simulink model "Discrete_EKF_2FMU"  (R2022a)
settings: Solver=ode23s  StartTime=0.0  StopTime=10  RelTol=1e-3
settings Model: Creator=au707539  LastModifiedBy=au707539
settings SolverCC: MaxZcPerStep=1
settings DebuggingCC: UnderSpecifiedDimensionMsg=warning

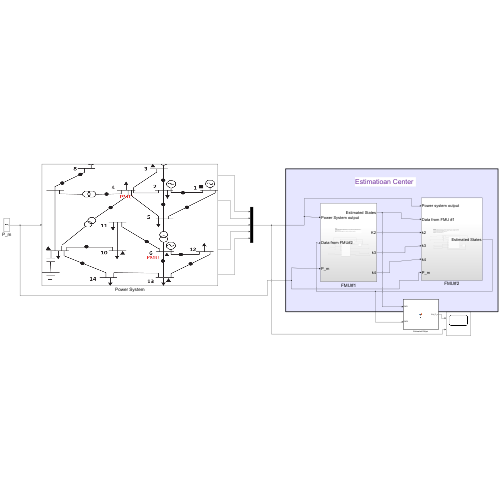
[thumbnail: Simulink's stored preview of the top-level diagram]
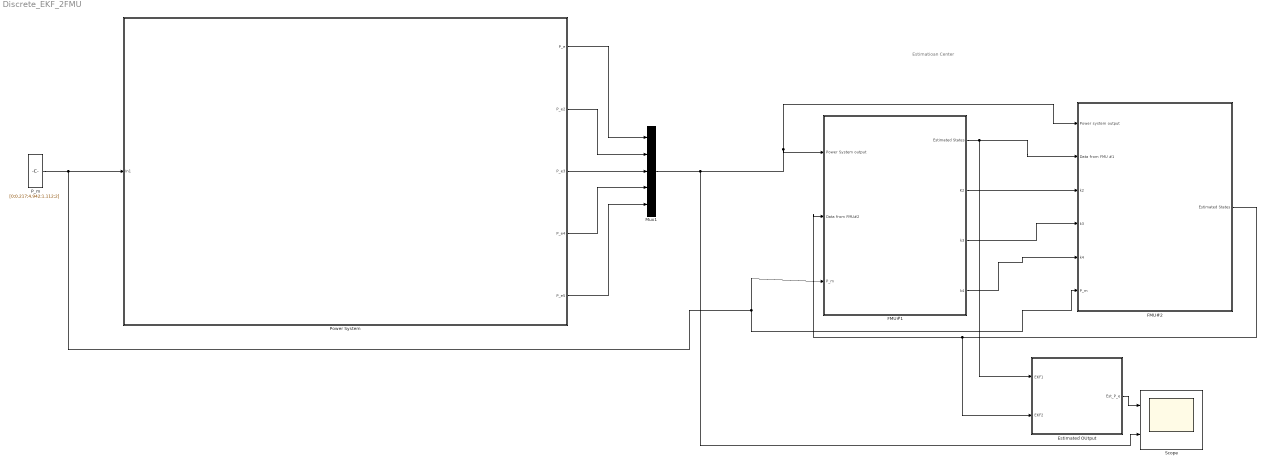
== system Discrete_EKF_2FMU ==
  note: Estimatioan Center
  Estimated OUtput : MATLAB Function  TreatAsAtomicUnit=on
  FMU#1 : Subsystem
  FMU#2 : Subsystem
  Mux1 : Mux  Inputs=5
  P_m : Constant  Value=[0;0.217;4.942;1.112;2]
  Power System : Subsystem
      mask Display: image('IEEE.png'); % Use "Edit Image" on toolstrip to change.
  Scope : Scope  NumInputPorts=2
  wires:
  P_m/1 -> FMU#1/3(P_m), FMU#2/6(P_m), Power System/1(In1)
  Mux1/1 -> Scope/2, FMU#2/1(Power system output), FMU#1/1(Power System output)
  Power System/1(P_e) -> Mux1/1
  Power System/2(P_e2) -> Mux1/2
  Power System/3(P_e3) -> Mux1/3
  Power System/4(P_e4) -> Mux1/4
  Power System/5(P_e5) -> Mux1/5
  FMU#1/1(Estimated States) -> Estimated OUtput/1(EKF1), FMU#2/2(Data from FMU #1)
  FMU#1/2(K2) -> FMU#2/3(k2)
  FMU#1/3(k3) -> FMU#2/4(k3)
  FMU#1/4(k4) -> FMU#2/5(k4)
  FMU#2/1(Estimated States) -> Estimated OUtput/2(EKF2), FMU#1/2(Data from FMU#2)
  Estimated OUtput/1(Est_P_e) -> Scope/1

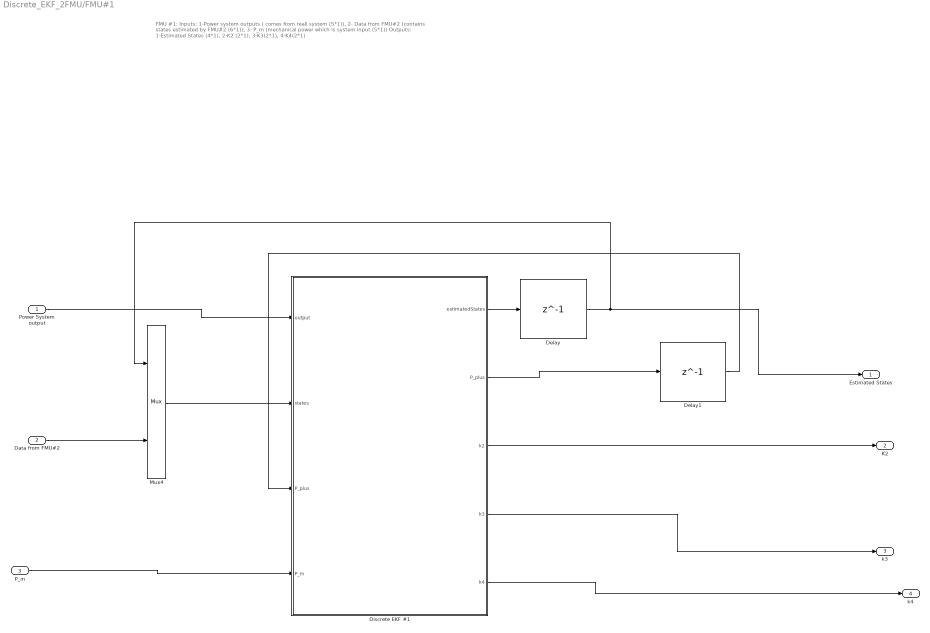
== system Discrete_EKF_2FMU/FMU#1 ==
  note: FMU #1:
      | Inputs: 1-Power system outputs ( comes from reall system (5*1)), 2- Data from FMU#2 (contains states estimated by FMU#2 (6*1)), 3- P_m (mechanical power which is system input (5*1))
      | Outputs: 1-Estimated States (4*1), 2-K2 (2*1), 3-K3(2*1), 4-K4(2*1)
  Power System output : Inport
  Data from FMU#2 : Inport  Port=2
  P_m : Inport  Port=3
  Delay : Delay  DelayLength=1  InitialCondition=[-0.152730000000000,-0.230910000000000,1,1]'  SampleTime=1e-4
  Delay1 : Delay  DelayLength=1  InitialCondition=0.01*eye(4)  SampleTime=1e-4
  Discrete EKF #1 : MATLAB Function  TreatAsAtomicUnit=on
  Mux4 : Mux  Inputs=2
  Estimated States : Outport
  K2 : Outport  Port=2
  k3 : Outport  Port=3
  k4 : Outport  Port=4
  wires:
  Discrete EKF #1/2(P_plus) -> Delay1/1
  Discrete EKF #1/1(estimatedStates) -> Delay/1
  Discrete EKF #1/3(k2) -> K2/1
  Power System output/1 -> Discrete EKF #1/1(output)
  Delay/1 -> Mux4/1, Estimated States/1
  Discrete EKF #1/4(k3) -> k3/1
  Mux4/1 -> Discrete EKF #1/2(states)
  Delay1/1 -> Discrete EKF #1/3("P_plus ")
  Discrete EKF #1/5(k4) -> k4/1
  P_m/1 -> Discrete EKF #1/4(P_m)
  Data from FMU#2/1 -> Mux4/2

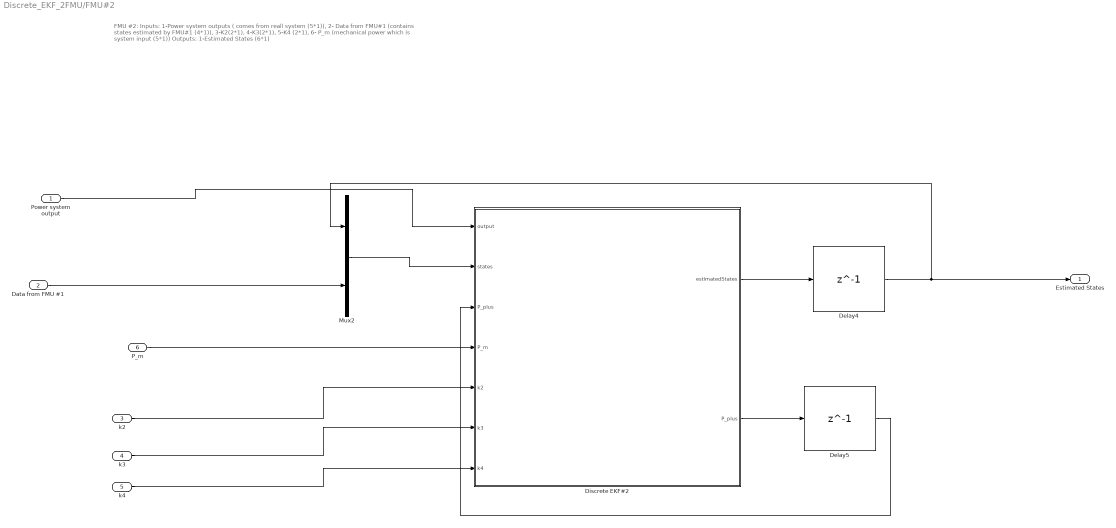
== system Discrete_EKF_2FMU/FMU#2 ==
  note: FMU #2:
      | Inputs: 1-Power system outputs ( comes from reall system (5*1)), 2- Data from FMU#1 (contains states estimated by FMU#1 (4*1)), 3-K2(2*1), 4-K3(2*1), 5-K4 (2*1), 6- P_m (mechanical power which is system input (5*1))
      | Outputs: 1-Estimated States (6*1)
  Power system output : Inport
  Data from FMU #1 : Inport  Port=2
  k2 : Inport  Port=3
  k3 : Inport  Port=4
  k4 : Inport  Port=5
  P_m : Inport  Port=6
  Delay4 : Delay  DelayLength=1  InitialCondition=[1.07618884220704,0.179610235169918,-0.222670000000000,1,1,1]'  SampleTime=1e-4
  Delay5 : Delay  DelayLength=1  InitialCondition=0.01*eye(6)  SampleTime=1e-4
  Discrete EKF#2 : MATLAB Function  TreatAsAtomicUnit=on
  Mux2 : Mux  Inputs=2
  Estimated States : Outport
  wires:
  Delay4/1 -> Mux2/1, Estimated States/1
  Data from FMU #1/1 -> Mux2/2
  Discrete EKF#2/1(estimatedStates) -> Delay4/1
  Delay5/1 -> Discrete EKF#2/3("P_plus ")
  Discrete EKF#2/2(P_plus) -> Delay5/1
  Mux2/1 -> Discrete EKF#2/2(states)
  P_m/1 -> Discrete EKF#2/4(P_m)
  Power system output/1 -> Discrete EKF#2/1(output)
  k4/1 -> Discrete EKF#2/7(k4)
  k2/1 -> Discrete EKF#2/5(k2)
  k3/1 -> Discrete EKF#2/6(k3)

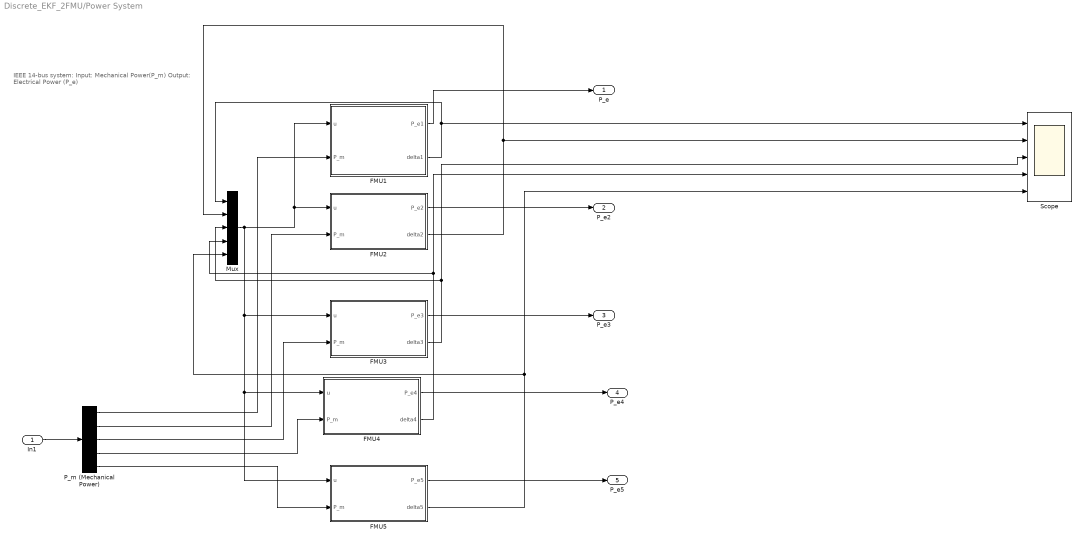
== system Discrete_EKF_2FMU/Power System ==
  note: IEEE 14-bus system:
      | Input: Mechanical Power(P_m)
      | Output: Electrical Power (P_e)
  In1 : Inport
  FMU1 : Subsystem
  FMU2 : Subsystem
  FMU3 : Subsystem
  FMU4 : Subsystem
  FMU5 : Subsystem
  Mux : Mux  Inputs=5
  P_m (Mechanical Power) : Demux  Outputs=5
  Scope : Scope  NumInputPorts=5
  P_e : Outport
  P_e2 : Outport  Port=2
  P_e3 : Outport  Port=3
  P_e4 : Outport  Port=4
  P_e5 : Outport  Port=5
  wires:
  FMU1/2(delta1) -> Scope/1, Mux/1
  FMU2/2(delta2) -> Scope/2, Mux/2
  In1/1 -> P_m (Mechanical Power)/1
  P_m (Mechanical Power)/1 -> FMU1/2(P_m)
  FMU1/1(P_e1) -> P_e/1
  P_m (Mechanical Power)/2 -> FMU2/2(P_m)
  FMU2/1(P_e2) -> P_e2/1
  P_m (Mechanical Power)/3 -> FMU3/2(P_m)
  FMU3/2(delta3) -> Scope/3, Mux/3
  FMU3/1(P_e3) -> P_e3/1
  P_m (Mechanical Power)/4 -> FMU4/2(P_m)
  FMU4/2(delta4) -> Scope/4, Mux/4
  FMU4/1(P_e4) -> P_e4/1
  P_m (Mechanical Power)/5 -> FMU5/2(P_m)
  FMU5/1(P_e5) -> P_e5/1
  FMU5/2(delta5) -> Mux/5, Scope/5
  Mux/1 -> FMU5/1(u), FMU4/1(u), FMU3/1(u), FMU2/1(u), FMU1/1(u)

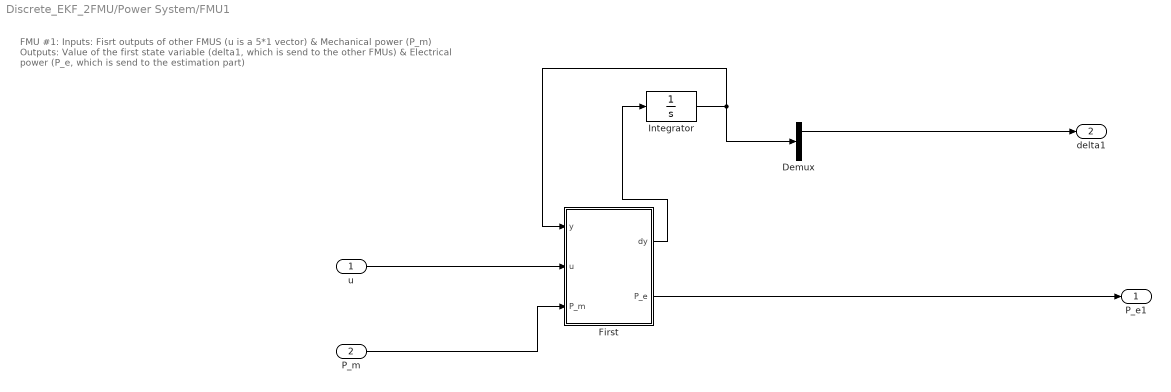
== system Discrete_EKF_2FMU/Power System/FMU1 ==
  note: FMU #1:
      | Inputs: Fisrt outputs of other FMUS (u is a 5*1 vector) & Mechanical power (P_m)
      | Outputs: Value of the first state variable (delta1, which is send to the other FMUs) & Electrical power (P_e, which is send to the estimation part)
  u : Inport
  P_m : Inport  Port=2
  Demux : Demux  Outputs=2
  First : MATLAB Function  TreatAsAtomicUnit=on
  Integrator : Integrator  InitialCondition=[1.0762;1]
  P_e1 : Outport
  delta1 : Outport  Port=2
  wires:
  u/1 -> First/2(u)
  Integrator/1 -> First/1(y), Demux/1
  First/1(dy) -> Integrator/1
  P_m/1 -> First/3(P_m)
  First/2(P_e) -> P_e1/1
  Demux/1 -> delta1/1

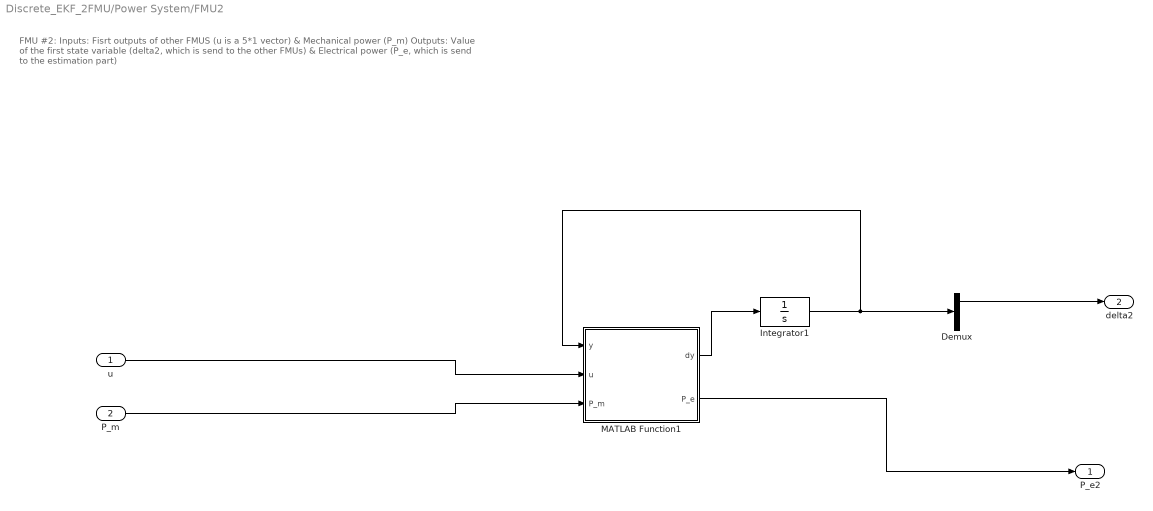
== system Discrete_EKF_2FMU/Power System/FMU2 ==
  note: FMU #2:
      | Inputs: Fisrt outputs of other FMUS (u is a 5*1 vector) & Mechanical power (P_m)
      | Outputs: Value of the first state variable (delta2, which is send to the other FMUs) & Electrical power (P_e, which is send to the estimation part)
  u : Inport
  P_m : Inport  Port=2
  Demux : Demux  Outputs=2
  Integrator1 : Integrator  InitialCondition=[0.1796;1]
  MATLAB Function1 : MATLAB Function  TreatAsAtomicUnit=on
  P_e2 : Outport
  delta2 : Outport  Port=2
  wires:
  P_m/1 -> MATLAB Function1/3(P_m)
  MATLAB Function1/1(dy) -> Integrator1/1
  u/1 -> MATLAB Function1/2(u)
  Integrator1/1 -> Demux/1, MATLAB Function1/1(y)
  Demux/1 -> delta2/1
  MATLAB Function1/2(P_e) -> P_e2/1

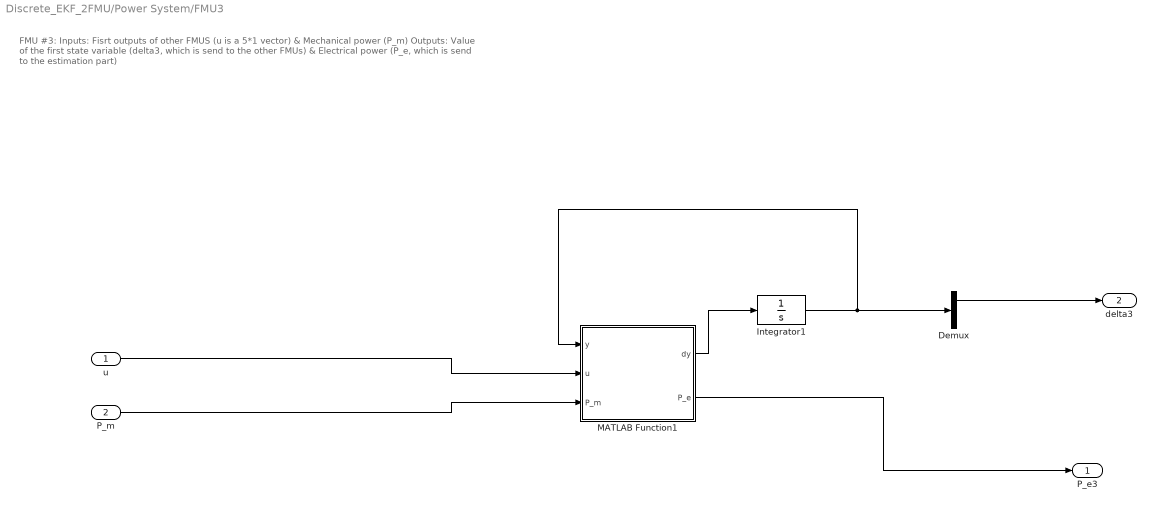
== system Discrete_EKF_2FMU/Power System/FMU3 ==
  note: FMU #3:
      | Inputs: Fisrt outputs of other FMUS (u is a 5*1 vector) & Mechanical power (P_m)
      | Outputs: Value of the first state variable (delta3, which is send to the other FMUs) & Electrical power (P_e, which is send to the estimation part)
  u : Inport
  P_m : Inport  Port=2
  Demux : Demux  Outputs=2
  Integrator1 : Integrator  InitialCondition=[-0.22267;1]
  MATLAB Function1 : MATLAB Function  TreatAsAtomicUnit=on
  P_e3 : Outport
  delta3 : Outport  Port=2
  wires:
  P_m/1 -> MATLAB Function1/3(P_m)
  MATLAB Function1/1(dy) -> Integrator1/1
  u/1 -> MATLAB Function1/2(u)
  Integrator1/1 -> Demux/1, MATLAB Function1/1(y)
  Demux/1 -> delta3/1
  MATLAB Function1/2(P_e) -> P_e3/1

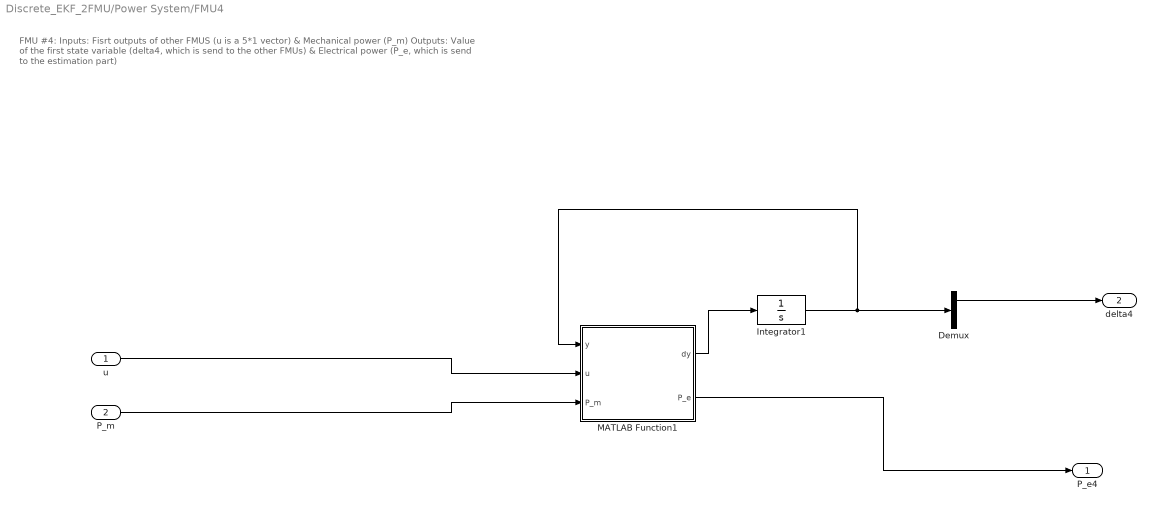
== system Discrete_EKF_2FMU/Power System/FMU4 ==
  note: FMU #4:
      | Inputs: Fisrt outputs of other FMUS (u is a 5*1 vector) & Mechanical power (P_m)
      | Outputs: Value of the first state variable (delta4, which is send to the other FMUs) & Electrical power (P_e, which is send to the estimation part)
  u : Inport
  P_m : Inport  Port=2
  Demux : Demux  Outputs=2
  Integrator1 : Integrator  InitialCondition=[-0.15273;1]
  MATLAB Function1 : MATLAB Function  TreatAsAtomicUnit=on
  P_e4 : Outport
  delta4 : Outport  Port=2
  wires:
  P_m/1 -> MATLAB Function1/3(P_m)
  MATLAB Function1/1(dy) -> Integrator1/1
  u/1 -> MATLAB Function1/2(u)
  Integrator1/1 -> Demux/1, MATLAB Function1/1(y)
  Demux/1 -> delta4/1
  MATLAB Function1/2(P_e) -> P_e4/1

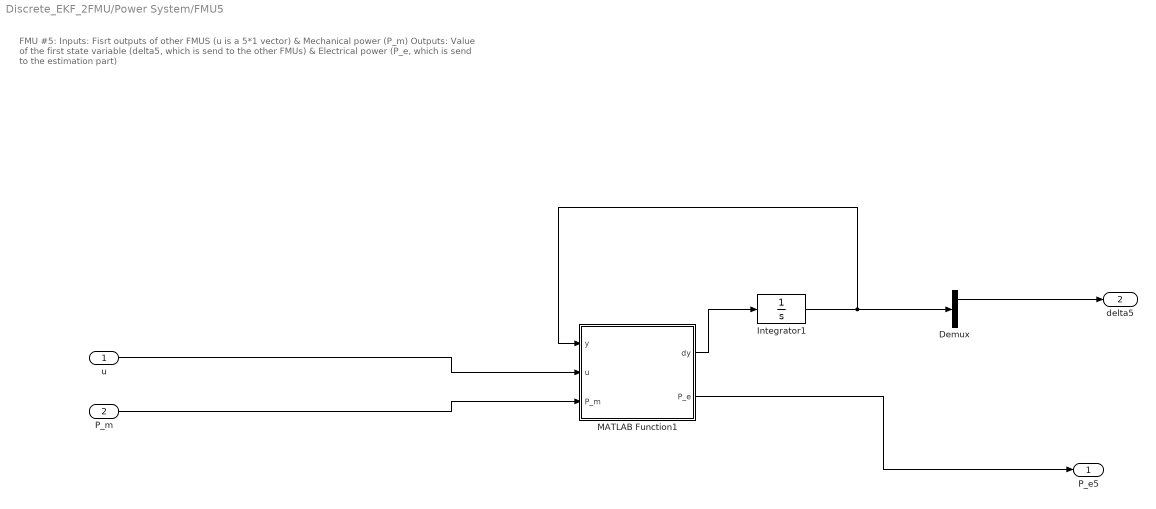
== system Discrete_EKF_2FMU/Power System/FMU5 ==
  note: FMU #5:
      | Inputs: Fisrt outputs of other FMUS (u is a 5*1 vector) & Mechanical power (P_m)
      | Outputs: Value of the first state variable (delta5, which is send to the other FMUs) & Electrical power (P_e, which is send to the estimation part)
  u : Inport
  P_m : Inport  Port=2
  Demux : Demux  Outputs=2
  Integrator1 : Integrator  InitialCondition=[-0.23091;1]
  MATLAB Function1 : MATLAB Function  TreatAsAtomicUnit=on
  P_e5 : Outport
  delta5 : Outport  Port=2
  wires:
  P_m/1 -> MATLAB Function1/3(P_m)
  MATLAB Function1/1(dy) -> Integrator1/1
  u/1 -> MATLAB Function1/2(u)
  Integrator1/1 -> Demux/1, MATLAB Function1/1(y)
  Demux/1 -> delta5/1
  MATLAB Function1/2(P_e) -> P_e5/1

== matlab function Discrete_EKF_2FMU/Power System/FMU2/MATLAB Function1 ==
  data: y input; u input; dy output; P_m input; P_e output
%% This function formulates the dynamic model of the second synchronous machine in IEEE-14 bus test system
%% y is the state vector related to this Genrator, u is vector of all generators angles (delta), and P-m is Mechanical power injected to this machine
%% dy is the derivative of y which is calculated in this function and P-e is the electrical power which is calculated in this function
function [dy,P_e] = fcn(y,u,P_m)
dy=zeros(2,1);
P_e=0;
%%%%%%%Generators and network parameters (they can be defined as global
%%%%%%%parameters because they are fixed for all generators)%%%%%%%%%%%
N_SG=5;
X_d=[0.898 1.05 1.05 1.25 1.25];
Vol_mag=[1.06 1.045 1.01 1.011981 1.049336 1.016012 1.07 1.09 1.032756 1.03177 1.04708 1.053428 1.046967 1.020701];
P_Gen=[2.32 0.4 0 0 0];
Q_Gen=[0 0.424 0 0 0];
VOl_mag_Gen=[Vol_mag(1) Vol_mag(2) Vol_mag(3) Vol_mag(6) Vol_mag(8)];
M=[3.52e-3 0.436e-3 0.436e-3 1.406e-4 1.406e-4];
D=[2 2 2 2 2];
Y=[0.1017-2.4199i, 0.0096+0.9097i, -0.0567+0.5006i, -0.0322+0.4973i, -0.0186+0.5531i; 0.0096+0.9097i, 0.1375-3.5521i, -0.0574+0.9568i, -0.0437+0.8608i, ...
    -0.0395+0.8903i; -0.0567+0.5006i, -0.0574+0.9568i, 0.2630-2.9134i, -0.0640+0.8148i, -0.0791+0.6968i; -0.0322+0.4973i, -0.0437+0.8608i, -0.0640+0.8148i,...
    0.1156-3.0762i, 0.0303+0.9547i; -0.0186+0.5531i, -0.0395+0.8903i, -0.0791+0.6968i, 0.0303+0.9547i, 0.1117-3.0513i];
% [v_r, v_i]=pol2cart(Degrre_Gen,Vol_mag_Gen);

E_abs=zeros(5,1);
for i=1:5
    %     delta0(i)=angle(VOl_mag_Gen(i)+Q_Gen(i).*X_d(i)./VOl_mag_Gen(i) + 1i*P_Gen(i).*X_d(i)./VOl_mag_Gen(i))+Degrre_Gen(i);
    E_abs(i)=abs(VOl_mag_Gen(i)+Q_Gen(i).*X_d(i)./VOl_mag_Gen(i) + 1i*P_Gen(i).*X_d(i)./VOl_mag_Gen(i));
end
%%%%%%%%%%%%%%%%%%%%%%%%%%
delta=u(1:5);
sum1=0; %% local parameter
for j=1:N_SG

    sum1=sum1+E_abs(2)*E_abs(j)*abs(Y(2,j))*cos(delta(2)-delta(j)-angle(Y(2,j))); % All angles in Radian
end
P_e=sum1;

P_e=sum1;  % Second output (which is send to the estimation part)

dy(1)=y(2); %first entry of the function output

dy(2) =(1/M(2))*(P_m-P_e-D(2)*y(2));  %Second entry of the function output

== matlab function Discrete_EKF_2FMU/Power System/FMU1/First ==
  data: y input; u input; dy output; P_m input; P_e output
%% This function formulates the dynamic model of the first synchronous machine in IEEE-14 bus test system
%% y is the state vector related to this Genrator, u is vector of all generators angles (delta), and P-m is Mechanical power injected to this machine
%% dy is the derivative of y which is calculated in this function and P-e is the electrical power which is calculated in this function
function [dy,P_e] = fcn(y,u,P_m) 
dy=zeros(2,1);

%%%%%%%Generators and network parameters (they can be defined as global
%%%%%%%parameters because they are fixed for all generators)%%%%%%%%%%%%%
N_SG=5;
X_d=[0.898 1.05 1.05 1.25 1.25];
Vol_mag=[1.06 1.045 1.01 1.011981 1.049336 1.016012 1.07 1.09 1.032756 1.03177 1.04708 1.053428 1.046967 1.020701];
P_Gen=[2.32 0.4 0 0 0];
Q_Gen=[0 0.424 0 0 0];
VOl_mag_Gen=[Vol_mag(1) Vol_mag(2) Vol_mag(3) Vol_mag(6) Vol_mag(8)];
M=[3.52e-3 0.436e-3 0.436e-3 1.406e-4 1.406e-4];
D=[2 2 2 2 2];
Y=[0.1017-2.4199i, 0.0096+0.9097i, -0.0567+0.5006i, -0.0322+0.4973i, -0.0186+0.5531i; 0.0096+0.9097i, 0.1375-3.5521i, -0.0574+0.9568i, -0.0437+0.8608i, ...
    -0.0395+0.8903i; -0.0567+0.5006i, -0.0574+0.9568i, 0.2630-2.9134i, -0.0640+0.8148i, -0.0791+0.6968i; -0.0322+0.4973i, -0.0437+0.8608i, -0.0640+0.8148i,...
    0.1156-3.0762i, 0.0303+0.9547i; -0.0186+0.5531i, -0.0395+0.8903i, -0.0791+0.6968i, 0.0303+0.9547i, 0.1117-3.0513i];
% [v_r, v_i]=pol2cart(Degrre_Gen,Vol_mag_Gen);

E_abs=zeros(5,1); %local parameter
for i=1:5
    %     delta0(i)=angle(VOl_mag_Gen(i)+Q_Gen(i).*X_d(i)./VOl_mag_Gen(i) + 1i*P_Gen(i).*X_d(i)./VOl_mag_Gen(i))+Degrre_Gen(i);
    E_abs(i)=abs(VOl_mag_Gen(i)+Q_Gen(i).*X_d(i)./VOl_mag_Gen(i) + 1i*P_Gen(i).*X_d(i)./VOl_mag_Gen(i));
end
%%%%%%%%%%%%%%%%%%%%%%%%%%
delta=u(1:5);
sum1=0; %% local parameter
for j=1:N_SG

    sum1=sum1+E_abs(1)*E_abs(j)*abs(Y(1,j))*cos(delta(1)-delta(j)-angle(Y(1,j))); % All angles in Radian
end

P_e=sum1;  % Second output (which is send to the estimation part)

dy(1)=y(2); %first entry of the function output

dy(2) =(1/M(1))*(P_m-P_e-D(1)*y(2)); %Second entry of the function output

== matlab function Discrete_EKF_2FMU/Power System/FMU4/MATLAB Function1 ==
  data: y input; u input; dy output; P_m input; P_e output
%% This function formulates the dynamic model of the fourth synchronous machine in IEEE-14 bus test system
%% y is the state vector related to this Genrator, u is vector of all generators angles (delta), and P-m is Mechanical power injected to this machine
%% dy is the derivative of y which is calculated in this function and P-e is the electrical power which is calculated in this function
function [dy,P_e] = fcn(y,u,P_m)
dy=zeros(2,1);
P_e=0;
%%%%%%%Generators and network parameters (they can be defined as global
%%%%%%%parameters because they are fixed for all generators)%%%%%%%%%%%
N_SG=5;
X_d=[0.898 1.05 1.05 1.25 1.25];
Vol_mag=[1.06 1.045 1.01 1.011981 1.049336 1.016012 1.07 1.09 1.032756 1.03177 1.04708 1.053428 1.046967 1.020701];
P_Gen=[2.32 0.4 0 0 0];
Q_Gen=[0 0.424 0 0 0];
VOl_mag_Gen=[Vol_mag(1) Vol_mag(2) Vol_mag(3) Vol_mag(6) Vol_mag(8)];
M=[3.52e-3 0.436e-3 0.436e-3 1.406e-4 1.406e-4];
D=[2 2 2 2 2];
Y=[0.1017-2.4199i, 0.0096+0.9097i, -0.0567+0.5006i, -0.0322+0.4973i, -0.0186+0.5531i; 0.0096+0.9097i, 0.1375-3.5521i, -0.0574+0.9568i, -0.0437+0.8608i, ...
    -0.0395+0.8903i; -0.0567+0.5006i, -0.0574+0.9568i, 0.2630-2.9134i, -0.0640+0.8148i, -0.0791+0.6968i; -0.0322+0.4973i, -0.0437+0.8608i, -0.0640+0.8148i,...
    0.1156-3.0762i, 0.0303+0.9547i; -0.0186+0.5531i, -0.0395+0.8903i, -0.0791+0.6968i, 0.0303+0.9547i, 0.1117-3.0513i];
% [v_r, v_i]=pol2cart(Degrre_Gen,Vol_mag_Gen);

E_abs=zeros(5,1);
for i=1:5
    %     delta0(i)=angle(VOl_mag_Gen(i)+Q_Gen(i).*X_d(i)./VOl_mag_Gen(i) + 1i*P_Gen(i).*X_d(i)./VOl_mag_Gen(i))+Degrre_Gen(i);
    E_abs(i)=abs(VOl_mag_Gen(i)+Q_Gen(i).*X_d(i)./VOl_mag_Gen(i) + 1i*P_Gen(i).*X_d(i)./VOl_mag_Gen(i));
end
%%%%%%%%%%%%%%%%%%%%%%%%%%
delta=u(1:5);
sum1=0; %% local parameter
for j=1:N_SG

    sum1=sum1+E_abs(4)*E_abs(j)*abs(Y(4,j))*cos(delta(4)-delta(j)-angle(Y(4,j))); % All angles in Radian
end

P_e=sum1;

P_e=sum1;  % Second output (which is send to the estimation part)

dy(1)=y(2); %first entry of the function output

dy(2) =(1/M(4))*(P_m-P_e-D(4)*y(2));  %Second entry of the function output

== matlab function Discrete_EKF_2FMU/Power System/FMU5/MATLAB Function1 ==
  data: y input; u input; dy output; P_m input; P_e output
%% This function formulates the dynamic model of the fifth synchronous machine in IEEE-14 bus test system
%% y is the state vector related to this Genrator, u is vector of all generators angles (delta), and P-m is Mechanical power injected to this machine
%% dy is the derivative of y which is calculated in this function and P-e is the electrical power which is calculated in this function
function [dy,P_e] = fcn(y,u,P_m)
dy=zeros(2,1);
P_e=0;
%%%%%%%Generators and network parameters (they can be defined as global
%%%%%%%parameters because they are fixed for all generators)%%%%%%%%%%%
N_SG=5;
X_d=[0.898 1.05 1.05 1.25 1.25];
Vol_mag=[1.06 1.045 1.01 1.011981 1.049336 1.016012 1.07 1.09 1.032756 1.03177 1.04708 1.053428 1.046967 1.020701];
P_Gen=[2.32 0.4 0 0 0];
Q_Gen=[0 0.424 0 0 0];
VOl_mag_Gen=[Vol_mag(1) Vol_mag(2) Vol_mag(3) Vol_mag(6) Vol_mag(8)];
M=[3.52e-3 0.436e-3 0.436e-3 1.406e-4 1.406e-4];
D=[2 2 2 2 2];
Y=[0.1017-2.4199i, 0.0096+0.9097i, -0.0567+0.5006i, -0.0322+0.4973i, -0.0186+0.5531i; 0.0096+0.9097i, 0.1375-3.5521i, -0.0574+0.9568i, -0.0437+0.8608i, ...
    -0.0395+0.8903i; -0.0567+0.5006i, -0.0574+0.9568i, 0.2630-2.9134i, -0.0640+0.8148i, -0.0791+0.6968i; -0.0322+0.4973i, -0.0437+0.8608i, -0.0640+0.8148i,...
    0.1156-3.0762i, 0.0303+0.9547i; -0.0186+0.5531i, -0.0395+0.8903i, -0.0791+0.6968i, 0.0303+0.9547i, 0.1117-3.0513i];
% [v_r, v_i]=pol2cart(Degrre_Gen,Vol_mag_Gen);

E_abs=zeros(5,1);
for i=1:5
    %     delta0(i)=angle(VOl_mag_Gen(i)+Q_Gen(i).*X_d(i)./VOl_mag_Gen(i) + 1i*P_Gen(i).*X_d(i)./VOl_mag_Gen(i))+Degrre_Gen(i);
    E_abs(i)=abs(VOl_mag_Gen(i)+Q_Gen(i).*X_d(i)./VOl_mag_Gen(i) + 1i*P_Gen(i).*X_d(i)./VOl_mag_Gen(i));
end
%%%%%%%%%%%%%%%%%%%%%%%%%%
delta=u(1:5);
sum1=0; %% local parameter
for j=1:N_SG

    sum1=sum1+E_abs(5)*E_abs(j)*abs(Y(5,j))*cos(delta(5)-delta(j)-angle(Y(5,j))); % All angles in Radian
end

P_e=sum1;

P_e=sum1;  % Second output (which is send to the estimation part)

dy(1)=y(2); %first entry of the function output

dy(2) =(1/M(5))*(P_m-P_e-D(5)*y(2));  %Second entry of the function output

== matlab function Discrete_EKF_2FMU/FMU#1/Discrete EKF #1 ==
  data: output input; estimatedStates output; P_plus output; states input; P_plus input; P_m input; k2 output; k3 output; k4 output
%% This function calculates the estimated states of the synchronous machines #4 and #5
%% Outputs are: estimatedStates (4*1), P_plus (updated covariance matix 4*4), k2 (second parameters of RungeKutta for 4th and 5th angles 2*1), k3 (third parameters of RungeKutta for 4th and 5th angles 2*1),
%% k4 (fourth parameters of RungeKutta for 4th and 5th angles 2*1). Inputs are: output (comes from power system 5*1), states(includes states of previous sample of this function + FMU#2 10*1),P_plus (updated covariance matrix of previous sample 4*4),
%% and P_m (Mechanical power which is input of power system 5*1)
function [estimatedStates,P_plus,k2,k3,k4] = fcn(output,states,P_plus,P_m)

%%% Initialization
delta_plus=zeros(5,1);
delta_plus(4:5,1)=states(1:2,:);
delta_plus(1:3,1)=states(5:7,1);
omega_plus=zeros(5,1);
omega_plus(1:3,1)=states(8:10,1);
omega_plus(4:5,1)=states(3:4,:);

sigma=1e-2; % variance
Q=sigma^2*eye(4); %Covariance matrix of process noise
R=sigma^2*eye(2); % Covariance matrix of measurement noise
Dt=1e-4; % DelatT, sample time for discretization

%%% Power system parameters %%%%%%%%%%%%
n=5; %Number of synchronous machines
X_d=[0.898 1.05 1.05 1.25 1.25];
Angle_rad=[0 -0.0871 -0.22267 -0.1785 -0.23091 -0.15273 -0.25161 -0.23091 -0.25853 -0.26223 -0.25897 -0.26645 -0.2671 -0.28018];%% Bus voltage phases (all are in rad)
Vol_mag=[1.06 1.045 1.01 1.011981 1.049336 1.016012 1.07 1.09 1.032756 1.03177 1.04708 1.053428 1.046967 1.020701];%% Bus voltage magnitudes
P_Gen=[2.32 0.4 0 0 0]; % Active power
Q_Gen=[0 0.424 0 0 0]; % Reactive Power
M=[3.52e-3 0.436e-3 0.436e-3 1.406e-4 1.406e-4];
D=[2 2 2 2 2];
VOl_mag_Gen=[Vol_mag(1) Vol_mag(2) Vol_mag(3) Vol_mag(6) Vol_mag(8)];

%%Calculating the phases and magnitudes of the generator voltages
E_abs=zeros(5,1);
for i=1:5
    E_abs(i)=abs(VOl_mag_Gen(i)+Q_Gen(i).*X_d(i)./VOl_mag_Gen(i) + 1i*P_Gen(i).*X_d(i)./VOl_mag_Gen(i));
end

% Reduced admittance matrix (all in p.u.)
Y=[0.1017-2.4199i, 0.0096+0.9097i, -0.0567+0.5006i, -0.0322+0.4973i, -0.0186+0.5531i; 0.0096+0.9097i, 0.1375-3.5521i, -0.0574+0.9568i, -0.0437+0.8608i, ...
    -0.0395+0.8903i; -0.0567+0.5006i, -0.0574+0.9568i, 0.2630-2.9134i, -0.0640+0.8148i, -0.0791+0.6968i; -0.0322+0.4973i, -0.0437+0.8608i, -0.0640+0.8148i,...
    0.1156-3.0762i, 0.0303+0.9547i; -0.0186+0.5531i, -0.0395+0.8903i, -0.0791+0.6968i, 0.0303+0.9547i, 0.1117-3.0513i];

%-------------------------------------------------------------------------------------------------------------------------------------
%% Time Update %%%%%%%%%%%%
%%% Obtaining the discrete form of the system model using RungeKutta method

f_delta=[zeros(n),eye(n)]; % delta.dot=f_delta*[delta;omega]
k1_delta=f_delta*[delta_plus;omega_plus].*Dt; % k1_delta=f(x)*Dt % f(x)=w

dk1_delta_delta=zeros(5); %partial derivative of k1_delta with respect to delta
dk1_delta_omega=eye(5); %partial derivative of k1_delta with respect to omega
P_e=zeros(5,1);
k1_omega=zeros(5,1);
for i=1:n

    sum1=0;
    for j=1:n

        sum1=sum1+E_abs(i)*E_abs(j)*abs(Y(i,j))*cos(delta_plus(i)-delta_plus(j)-angle(Y(i,j))); % All angles in Radian
    end
    P_e(i)=sum1;

    k1_omega(i)=(1/M(i))*(P_m(i)-P_e(i)-D(i)*omega_plus(i))*Dt; %k1_omega=f(x)*Dt %f(x)=(1/M)*(P_m-P_e-Dw)
end

dk1_omega_delta=zeros(5); %partial derivative of k1_omega respect to delta
for j=1:5 % j represents the number of row
    for i=1:5 % i represents the number of column
        if i==j
            sum=0;
            for k=1:5 % k is counter 
                if k~=j
                    sum=sum+(Dt/M(j))*(E_abs(j)*E_abs(k)*abs(Y(j,k))*sin(delta_plus(j)-delta_plus(k)-angle(Y(j,k))));
                else
                    sum=sum;
                end          
            end
            dk1_omega_delta(j,i)=sum;
        else
            dk1_omega_delta(j,i)=-(Dt/M(j))*E_abs(j)*E_abs(i)*abs(Y(j,i))*sin(delta_plus(j)-delta_plus(i)-angle(Y(j,i)));
        end
    end
end

dk1_omega_omega=Dt.*diag(-D./M); %partial derivative of k1_omega respect to omega

k2_delta=(f_delta*([delta_plus;omega_plus]+[k1_delta;k1_omega]./2)).*Dt; %k2_delta=f(x+k1w/2)*Dt %
dk2_delta_delta=(Dt/2).*dk1_omega_delta;  % partial derivative of k2_delta respect to delta
dk2_delta_omega=Dt.*eye(5)+(Dt/2).*dk1_omega_omega; % Partial derivative of k2_delta respect to omega

k2_omega=zeros(5,1);
for i=1:n

    sum1=0;
    for j=1:n

        sum1=sum1+E_abs(i)*E_abs(j)*abs(Y(i,j))*cos((delta_plus(i)+k1_delta(i)/2)-(delta_plus(j)+k1_delta(j)/2)-angle(Y(i,j))); % All angles in Radian
    end
    P_e(i)=sum1;

    k2_omega(i)=(1/M(i))*(P_m(i)-P_e(i)-D(i)*(omega_plus(i)+k1_omega(i)/2))*Dt; %k2_omega=f(x+k1/2)*Dt
end
dP_k1=zeros(5);
for j=1:5 % j represents the number of row
    for i=1:5 % i represents the number of column
        if i==j
            sum=0;
            for k=1:5 % k is counter 
                if k~=j
                    sum=sum+(Dt/M(j))*E_abs(j)*E_abs(k)*abs(Y(j,k))*...
                        sin((delta_plus(j)+k1_delta(j)/2)-(delta_plus(k)+k1_delta(k)/2)-angle(Y(j,k)));
                else
                    sum=sum;
                end          
            end
            dP_k1(j,i)=sum; %% partial derivative P_e(delta+k1_delta/2) which apears in k2_omega
        else
            dP_k1(j,i)=-(Dt/M(j))*E_abs(j)*E_abs(i)*abs(Y(j,i))*...
                sin((delta_plus(j)+k1_delta(j)/2)-(delta_plus(i)+k1_delta(i)/2)-angle(Y(j,i)));
        end
    end
end

dk2_omega_omega=dP_k1*(1/2)*dk1_delta_omega-diag(Dt*D./M)-(1/2)*diag(Dt*D./M)*dk1_omega_omega;  %partial derivative of k2_omega respect to omega
dk2_omega_delta=dP_k1*(eye(5)+(1/2)*dk1_delta_delta)-(1/2)*diag(Dt*D./M)*dk1_omega_delta;  %partial derivative of k2_omega respect to delta

k3_delta=(f_delta*([delta_plus;omega_plus]+[k2_delta;k2_omega]./2)).*Dt; %k3_delta=f(x+k2w/2)*Dt
dk3_delta_delta=(Dt/2)*dk2_omega_delta;  %partial derivative of k3_delta respect to delta
dk3_delta_omega=Dt.*eye(5)+(Dt/2).*dk2_omega_omega;  %partial derivative of k3_delta respect to omega
k3_omega=zeros(5,1);
for i=1:n

    sum1=0;
    for j=1:n

        sum1=sum1+E_abs(i)*E_abs(j)*abs(Y(i,j))*cos((delta_plus(i)+k2_delta(i)/2)-(delta_plus(j)+k2_delta(j)/2)-angle(Y(i,j))); % All angles in Radian
    end
    P_e(i)=sum1;

    k3_omega(i)=(1/M(i))*(P_m(i)-P_e(i)-D(i)*(omega_plus(i)+k2_omega(i)/2))*Dt; %k3_omega=f(x+k2/2)*Dt
end

dP_k2=zeros(5);
for j=1:5 % j represents the number of row
    for i=1:5 % i represents the number of column
        if i==j
            sum=0;
            for k=1:5 % k is counter 
                if k~=j
                    sum=sum+(Dt/M(j))*E_abs(j)*E_abs(k)*abs(Y(j,k))*...
                        sin((delta_plus(j)+k2_delta(j)/2)-(delta_plus(k)+k2_delta(k)/2)-angle(Y(j,k)));
                else
                    sum=sum;
                end          
            end
            dP_k2(j,i)=sum; %% partial derivative P_e(delta+k2_delta/2) which apears in k3_omega
        else
            dP_k2(j,i)=-(Dt/M(j))*E_abs(j)*E_abs(i)*abs(Y(j,i))*...
                sin((delta_plus(j)+k2_delta(j)/2)-(delta_plus(i)+k2_delta(i)/2)-angle(Y(j,i)));
        end
    end
end

dk3_omega_delta=dP_k2*(eye(5)+(1/2)*dk2_delta_delta)-diag((Dt*D)./(2*M))*dk2_omega_delta;  %partial derivative of k3_omega respect to delta
dk3_omega_omega=dP_k2*(1/2)*dk2_delta_omega-diag(Dt*D./M)-diag((Dt*D)./(2*M))*dk2_omega_omega;  %partial derivative of k3_omega respect to omega

k4_delta=(f_delta*([delta_plus;omega_plus]+[k3_delta;k3_omega])).*Dt; %k4_delta=f(x+k3w)*Dt

dk4_delta_delta=Dt*dk3_omega_delta;    %partial derivative of k4_delta respect to delta
dk4_delta_omega=Dt*(eye(5)+dk3_omega_omega);  %partial derivative of k4_delta respect to omega

k4_omega=zeros(5,1);
for i=1:n

    sum1=0;
    for j=1:n

        sum1=sum1+E_abs(i)*E_abs(j)*abs(Y(i,j))*cos((delta_plus(i)+k3_delta(i))-(delta_plus(j)+k3_delta(j))-angle(Y(i,j))); % All angles in Radian
    end
    P_e(i)=sum1;

    k4_omega(i)=(1/M(i))*(P_m(i)-P_e(i)-D(i)*(omega_plus(i)+k3_omega(i)))*Dt; %k4_omega=f(x+k3)*Dt
end
dP_k3=zeros(5);
for j=1:5 % j represents the number of row
    for i=1:5 % i represents the number of column
        if i==j
            sum=0;
            for k=1:5 % k is counter 
                if k~=j
                    sum=sum+(Dt/M(j))*E_abs(j)*E_abs(k)*abs(Y(j,k))*...
                        sin((delta_plus(j)+k3_delta(j))-(delta_plus(k)+k3_delta(k))-angle(Y(j,k)));
                else
                    sum=sum;
                end          
            end
            dP_k3(j,i)=sum; %% partial derivative P_e(delta+k2_delta/2) which apears in k3_omega
        else
            dP_k3(j,i)=-(Dt/M(j))*E_abs(j)*E_abs(i)*abs(Y(j,i))*...
                sin((delta_plus(j)+k3_delta(j))-(delta_plus(i)+k3_delta(i))-angle(Y(j,i)));
        end
    end
end

dk4_omega_delta=dP_k3*(eye(5)+dk3_delta_delta)-diag((Dt*D)./M)*dk3_omega_delta;   %partial derivative of k4_omega respect to delta
dk4_omega_omega=dP_k3*dk3_delta_omega-diag(Dt*D./M)-diag((Dt*D)./M)*dk3_omega_omega;   %partial derivative of k4_omega respect to omega


%%% Structuring partial derivative matrices: F & L, 


F=eye(4)+(1/6).*[dk1_delta_delta(4:5,4:5)+2.*dk2_delta_delta(4:5,4:5)+2*dk3_delta_delta(4:5,4:5)+dk4_delta_delta(4:5,4:5),dk1_delta_omega(4:5,4:5)+2.*dk2_delta_omega(4:5,4:5)+2*dk3_delta_omega(4:5,4:5)+dk4_delta_omega(4:5,4:5);...
    dk1_omega_delta(4:5,4:5)+2.*dk2_omega_delta(4:5,4:5)+2*dk3_omega_delta(4:5,4:5)+dk4_omega_delta(4:5,4:5),dk1_omega_omega(4:5,4:5)+2.*dk2_omega_omega(4:5,4:5)+2*dk3_omega_omega(4:5,4:5)+dk4_omega_omega(4:5,4:5)];

L=eye(4);
%% Prediction:

delta_=delta_plus+(1/6).*(k1_delta+2*k2_delta+2*k3_delta+k4_delta); % all deltas should be calculated

omega_=omega_plus+(1/6).*(k1_omega+2*k2_omega+2*k3_omega+k4_omega);
P_=F*P_plus*F'+L*Q*L';

%% Measurement Update:
%%% Structuring partial derivative matrices H & V
C=zeros(2);
for j=4:5 % j stands for number of row
    for i=4:5 % i stands for number of column
        if i==j
            sum=0;
            for k=1:5
                if k~=j
                    sum=sum-(E_abs(j)*E_abs(k)*abs(Y(j,k))*sin(delta_plus(j)-delta_plus(k)-angle(Y(j,k))));
                else
                    sum=sum;
                end          
            C(j-3,i-3)=sum;
            end
        else
            C(j-3,i-3)=E_abs(j)*E_abs(i)*abs(Y(j,i))*sin(delta_plus(j)-delta_plus(i)-angle(Y(j,i)));
        end
    end
end
H=[C,zeros(2)];
V=eye(2);

%%% Correction:
estimatedOutput=zeros(2,1);
for i=4:5
    sum1=0;
    for j=1:5

        sum1=sum1+E_abs(i)*E_abs(j)*abs(Y(i,j))*cos(delta_(i)-delta_(j)-angle(Y(i,j))); % All angles in Radian
    end
    estimatedOutput(i-3)=sum1;
end

K_gain=P_*H'*(H*P_*H'+V*R*V')^-1;  % Calculating kalman gain
estimatedStates=[delta_(4:5);omega_(4:5)]+K_gain*(output(4:5)-estimatedOutput); % estimated states (outputs of this function)
P_plus=(eye(4)-K_gain*H)*P_;   % Updating estimation error covariance matrix (output of this function)
% 2nd, 3rd, and 4th Runge Kutta parameters for 4th and 5th angles
k2=[k2_delta(4,1);k2_delta(5,1)];
k3=[k3_delta(4,1);k3_delta(5,1)];
k4=[k4_delta(4,1);k4_delta(5,1)];

== matlab function Discrete_EKF_2FMU/Estimated OUtput ==
  data: EKF1 input; Est_P_e output; EKF2 input
function Est_P_e = fcn(EKF1,EKF2)
delta=zeros(5,1);
delta(1:3,1)=EKF2(1:3,1);
delta(4:5,1)=EKF1(1:2,1);
Y=[0.1017-2.4199i, 0.0096+0.9097i, -0.0567+0.5006i, -0.0322+0.4973i, -0.0186+0.5531i; 0.0096+0.9097i, 0.1375-3.5521i, -0.0574+0.9568i, -0.0437+0.8608i, ...
    -0.0395+0.8903i; -0.0567+0.5006i, -0.0574+0.9568i, 0.2630-2.9134i, -0.0640+0.8148i, -0.0791+0.6968i; -0.0322+0.4973i, -0.0437+0.8608i, -0.0640+0.8148i,...
    0.1156-3.0762i, 0.0303+0.9547i; -0.0186+0.5531i, -0.0395+0.8903i, -0.0791+0.6968i, 0.0303+0.9547i, 0.1117-3.0513i];

X_d=[0.898 1.05 1.05 1.25 1.25];
Vol_mag=[1.06 1.045 1.01 1.011981 1.049336 1.016012 1.07 1.09 1.032756 1.03177 1.04708 1.053428 1.046967 1.020701];%% Bus voltage magnitudes
P_Gen=[2.32 0.4 0 0 0]; % Active power
Q_Gen=[0 0.424 0 0 0]; % Reactive Power
VOl_mag_Gen=[Vol_mag(1) Vol_mag(2) Vol_mag(3) Vol_mag(6) Vol_mag(8)];


%%Calculating the phases and magnitudes of the generator voltages
E_abs=zeros(5,1);
for i=1:5
%     delta0(i)=angle(VOl_mag_Gen(i)+Q_Gen(i).*X_d(i)./VOl_mag_Gen(i) + 1i*P_Gen(i).*X_d(i)./VOl_mag_Gen(i))+Phase_Gen(i);
    E_abs(i)=abs(VOl_mag_Gen(i)+Q_Gen(i).*X_d(i)./VOl_mag_Gen(i) + 1i*P_Gen(i).*X_d(i)./VOl_mag_Gen(i));
end
Est_P_e=zeros(5,1);
for i=1:5
    sum1=0;
    for j=1:5

        sum1=sum1+E_abs(i)*E_abs(j)*abs(Y(i,j))*cos(delta(i)-delta(j)-angle(Y(i,j))); % All angles in Radian
    end
    Est_P_e(i,1)=sum1;
end

== matlab function Discrete_EKF_2FMU/FMU#2/Discrete EKF#2 ==
  data: output input; estimatedStates output; P_plus output; states input; P_plus input; P_m input; k2 input; k3 input; k4 input
%% This function calculates the estimated states of the synchronous machines #1, #2 and #3
%% Outputs are: estimatedStates (6*1), P_plus (updated covariance matix 6*6), Inputs are: output (comes from power system 5*1), states(includes states of previous sample of this function + FMU#1 (10*1)),P_plus (updated covariance matrix of previous sample 6*6),
%% , P_m (Mechanical power which is input of power system 5*1), k2, k3, and k4 (all come from FMU#1 with size 2*1)
function [estimatedStates,P_plus] = fcn(output,states,P_plus,P_m,k2,k3,k4)

%%% Initialization
delta_plus=zeros(5,1);
delta_plus(1:3,1)=states(1:3,:);
delta_plus(4:5,1)=states(7:8,:);
omega_plus=states(4:6,:);
sigma=1e-2; % variance
Q=sigma^2*eye(6); %Covariance matrix of process noise
R=sigma^2*eye(3); % Covariance matrix of measurement noise
n=5; %Number of synchronous machines
Dt=1e-4; % DelatT, sample time for discretization
X_d=[0.898 1.05 1.05 1.25 1.25];
Angle_rad=[0 -0.0871 -0.22267 -0.1785 -0.23091 -0.15273 -0.25161 -0.23091 -0.25853 -0.26223 -0.25897 -0.26645 -0.2671 -0.28018];%% Bus voltage phases (all are in rad)
Vol_mag=[1.06 1.045 1.01 1.011981 1.049336 1.016012 1.07 1.09 1.032756 1.03177 1.04708 1.053428 1.046967 1.020701];%% Bus voltage magnitudes
P_Gen=[2.32 0.4 0 0 0]; % Active power
Q_Gen=[0 0.424 0 0 0]; % Reactive Power
VOl_mag_Gen=[Vol_mag(1) Vol_mag(2) Vol_mag(3) Vol_mag(6) Vol_mag(8)];
Phase_Gen=[Angle_rad(1) Angle_rad(2) Angle_rad(3) Angle_rad(6) Angle_rad(8)];
% [v_r, v_i]=pol2cart(Degrre_Gen,Vol_mag_Gen);

%%Calculating the phases and magnitudes of the generator voltages
E_abs=zeros(5,1);
for i=1:5
%     delta0(i)=angle(VOl_mag_Gen(i)+Q_Gen(i).*X_d(i)./VOl_mag_Gen(i) + 1i*P_Gen(i).*X_d(i)./VOl_mag_Gen(i))+Phase_Gen(i);
    E_abs(i)=abs(VOl_mag_Gen(i)+Q_Gen(i).*X_d(i)./VOl_mag_Gen(i) + 1i*P_Gen(i).*X_d(i)./VOl_mag_Gen(i));
end

% Reduced admittance matrix (all in p.u.)
Y=[0.1017-2.4199i, 0.0096+0.9097i, -0.0567+0.5006i, -0.0322+0.4973i, -0.0186+0.5531i; 0.0096+0.9097i, 0.1375-3.5521i, -0.0574+0.9568i, -0.0437+0.8608i, ...
    -0.0395+0.8903i; -0.0567+0.5006i, -0.0574+0.9568i, 0.2630-2.9134i, -0.0640+0.8148i, -0.0791+0.6968i; -0.0322+0.4973i, -0.0437+0.8608i, -0.0640+0.8148i,...
    0.1156-3.0762i, 0.0303+0.9547i; -0.0186+0.5531i, -0.0395+0.8903i, -0.0791+0.6968i, 0.0303+0.9547i, 0.1117-3.0513i];

%---------------------------------------------------------------------------------------------------------------------------------------
M=[3.52e-3 0.436e-3 0.436e-3 1.406e-4 1.406e-4];
D=[2 2 2 2 2];
%%% Continoues time functions
f_delta=[zeros(3),eye(3)]; % delta.dot=f_delta*[delta;omega]
f_deltaa=[zeros(5),eye(5)];

%% Time Update 
k1_delta=f_deltaa*[delta_plus;omega_plus;states(9,1);states(10)].*Dt; % k1_delta=f(x)*Dt % f(x)=w


dk1_delta_delta=zeros(3); %partial derivative of k1_delta with respect to delta
dk1_delta_omega=eye(3); %partial derivative of k1_delta with respect to omega
P_e=zeros(3,1);
k1_omega=zeros(3,1);
for i=1:3

    sum1=0;
    for j=1:n

        sum1=sum1+E_abs(i)*E_abs(j)*abs(Y(i,j))*cos(delta_plus(i)-delta_plus(j)-angle(Y(i,j))); % All angles in Radian
    end
    P_e(i)=sum1;

    k1_omega(i)=(1/M(i))*(P_m(i)-P_e(i)-D(i)*omega_plus(i))*Dt; %k1_omega=f(x)*Dt %f(x)=(1/M)*(P_m-P_e-Dw)
end
dk1_omega_delta=zeros(3);
for j=1:3 % j represents the number of row
    for i=1:3 % i represents the number of column
        if i==j
            sum=0;
            for k=1:5 % k is counter 
                if k~=j
                    sum=sum+(Dt/M(j))*(E_abs(j)*E_abs(k)*abs(Y(j,k))*sin(delta_plus(j)-delta_plus(k)-angle(Y(j,k))));
                else
                    sum=sum;
                end          
            end
            dk1_omega_delta(j,i)=sum;
        else
            dk1_omega_delta(j,i)=-(Dt/M(j))*E_abs(j)*E_abs(i)*abs(Y(j,i))*sin(delta_plus(j)-delta_plus(i)-angle(Y(j,i)));
        end
    end
end

dk1_omega_omega=Dt.*diag(-D(1:3)./M(1:3));
k2_delta=zeros(5,1);
k2_delta(1:3,1)=(f_delta*([delta_plus(1:3,:);omega_plus]+[k1_delta(1:3,:);k1_omega]./2)).*Dt; %k2_delta=f(x+k1w/2)*Dt %
k2_delta(4,1)=k2(1,1);
k2_delta(5,1)=k2(2,1);

dk2_delta_delta=(Dt/2).*dk1_omega_delta;
dk2_delta_omega=Dt.*eye(3)+(Dt/2).*dk1_omega_omega;
k2_omega=zeros(3,1);
for i=1:3

    sum1=0;
    for j=1:n

        sum1=sum1+E_abs(i)*E_abs(j)*abs(Y(i,j))*cos((delta_plus(i)+k1_delta(i)/2)-(delta_plus(j)+k1_delta(j)/2)-angle(Y(i,j))); % All angles in Radian
    end
    P_e(i)=sum1;

    k2_omega(i)=(1/M(i))*(P_m(i)-P_e(i)-D(i)*(omega_plus(i)+k1_omega(i)/2))*Dt; %k2_omega=f(x+k1/2)*Dt
end
dP_k1=zeros(3);
for j=1:3 % j represents the number of row
    for i=1:3 % i represents the number of column
        if i==j
            sum=0;
            for k=1:5 % k is counter 
                if k~=j
                    sum=sum+(Dt/M(j))*E_abs(j)*E_abs(k)*abs(Y(j,k))*...
                        sin((delta_plus(j)+k1_delta(j)/2)-(delta_plus(k)+k1_delta(k)/2)-angle(Y(j,k)));
                else
                    sum=sum;
                end          
            end
            dP_k1(j,i)=sum; %% partial derivative P_e(delta+k1_delta/2) which apears in k2_omega
        else
            dP_k1(j,i)=-(Dt/M(j))*E_abs(j)*E_abs(i)*abs(Y(j,i))*...
                sin((delta_plus(j)+k1_delta(j)/2)-(delta_plus(i)+k1_delta(i)/2)-angle(Y(j,i)));
        end
    end
end

dk2_omega_omega=dP_k1*(1/2)*dk1_delta_omega-diag(Dt*D(1:3)./M(1:3))-(1/2)*diag(Dt*D(1:3)./M(1:3))*dk1_omega_omega;
dk2_omega_delta=dP_k1*(eye(3)+(1/2)*dk1_delta_delta)-(1/2)*diag(Dt*D(1:3)./M(1:3))*dk1_omega_delta;

k3_delta=zeros(5,1);
k3_delta(1:3,1)=(f_delta*([delta_plus(1:3,:);omega_plus]+[k2_delta(1:3,:);k2_omega]./2)).*Dt; %k3_delta=f(x+k2w/2)*Dt
k3_delta(4,1)=k3(1,1);
k3_delta(5,1)=k3(2,1);

dk3_delta_delta=(Dt/2)*dk2_omega_delta;
dk3_delta_omega=Dt.*eye(3)+(Dt/2).*dk2_omega_omega;
k3_omega=zeros(3,1);
for i=1:3

    sum1=0;
    for j=1:n

        sum1=sum1+E_abs(i)*E_abs(j)*abs(Y(i,j))*cos((delta_plus(i)+k2_delta(i)/2)-(delta_plus(j)+k2_delta(j)/2)-angle(Y(i,j))); % All angles in Radian
    end
    P_e(i)=sum1;

    k3_omega(i)=(1/M(i))*(P_m(i)-P_e(i)-D(i)*(omega_plus(i)+k2_omega(i)/2))*Dt; %k3_omega=f(x+k2/2)*Dt
end

dP_k2=zeros(3);
for j=1:3 % j represents the number of row
    for i=1:3 % i represents the number of column
        if i==j
            sum=0;
            for k=1:5 % k is counter 
                if k~=j
                    sum=sum+(Dt/M(j))*E_abs(j)*E_abs(k)*abs(Y(j,k))*...
                        sin((delta_plus(j)+k2_delta(j)/2)-(delta_plus(k)+k2_delta(k)/2)-angle(Y(j,k)));
                else
                    sum=sum;
                end          
            end
            dP_k2(j,i)=sum; %% partial derivative P_e(delta+k2_delta/2) which apears in k3_omega
        else
            dP_k2(j,i)=-(Dt/M(j))*E_abs(j)*E_abs(i)*abs(Y(j,i))*...
                sin((delta_plus(j)+k2_delta(j)/2)-(delta_plus(i)+k2_delta(i)/2)-angle(Y(j,i)));
        end
    end
end

dk3_omega_delta=dP_k2*(eye(3)+(1/2)*dk2_delta_delta)-diag((Dt*D(1:3))./(2*M(1:3)))*dk2_omega_delta;
dk3_omega_omega=dP_k2*(1/2)*dk2_delta_omega-diag(Dt*D(1:3)./M(1:3))-diag((Dt*D(1:3))./(2*M(1:3)))*dk2_omega_omega;

k4_delta=zeros(5,1);
k4_delta(1:3,:)=(f_delta*([delta_plus(1:3);omega_plus]+[k3_delta(1:3,1);k3_omega])).*Dt; %k4_delta=f(x+k3w)*Dt
k4_delta(4,1)=k4(1,1);
k4_delta(5,1)=k4(2,1);

dk4_delta_delta=Dt*dk3_omega_delta;
dk4_delta_omega=Dt*(eye(3)+dk3_omega_omega);

k4_omega=zeros(3,1);
for i=1:3

    sum1=0;
    for j=1:n

        sum1=sum1+E_abs(i)*E_abs(j)*abs(Y(i,j))*cos((delta_plus(i)+k3_delta(i))-(delta_plus(j)+k3_delta(j))-angle(Y(i,j))); % All angles in Radian
    end
    P_e(i)=sum1;

    k4_omega(i)=(1/M(i))*(P_m(i)-P_e(i)-D(i)*(omega_plus(i)+k3_omega(i)))*Dt; %k4_omega=f(x+k3)*Dt
end
dP_k3=zeros(3);
for j=1:3 % j represents the number of row
    for i=1:3 % i represents the number of column
        if i==j
            sum=0;
            for k=1:5 % k is counter 
                if k~=j
                    sum=sum+(Dt/M(j))*E_abs(j)*E_abs(k)*abs(Y(j,k))*...
                        sin((delta_plus(j)+k3_delta(j))-(delta_plus(k)+k3_delta(k))-angle(Y(j,k)));
                else
                    sum=sum;
                end          
            end
            dP_k3(j,i)=sum; %% partial derivative P_e(delta+k2_delta/2) which apears in k3_omega
        else
            dP_k3(j,i)=-(Dt/M(j))*E_abs(j)*E_abs(i)*abs(Y(j,i))*...
                sin((delta_plus(j)+k3_delta(j))-(delta_plus(i)+k3_delta(i))-angle(Y(j,i)));
        end
    end
end

dk4_omega_delta=dP_k3*(eye(3)+dk3_delta_delta)-diag((Dt*D(1:3))./M(1:3))*dk3_omega_delta;
dk4_omega_omega=dP_k3*dk3_delta_omega-diag(Dt*D(1:3)./M(1:3))-diag((Dt*D(1:3))./M(1:3))*dk3_omega_omega;


%%% Structuring partial derivative matrices: F & L, 


F=eye(2*3)+(1/6).*[dk1_delta_delta+2.*dk2_delta_delta+2*dk3_delta_delta+dk4_delta_delta,dk1_delta_omega+2.*dk2_delta_omega+2*dk3_delta_omega+dk4_delta_omega;...
    dk1_omega_delta+2.*dk2_omega_delta+2*dk3_omega_delta+dk4_omega_delta,dk1_omega_omega+2.*dk2_omega_omega+2*dk3_omega_omega+dk4_omega_omega];

L=eye(6);
%% Prediction:

delta_=delta_plus+(1/6).*(k1_delta+2*k2_delta+2*k3_delta+k4_delta);

omega_=omega_plus+(1/6).*(k1_omega+2*k2_omega+2*k3_omega+k4_omega);........
P_=F*P_plus*F'+L*Q*L';

%% Measurement Update:
%%% Structuring partial derivative matrices H & V
C=zeros(3);
for j=1:3 % j stands for number of row
    for i=1:3 % i stands for number of column
        if i==j
            sum=0;
            for k=1:5
                if k~=j
                    sum=sum-(E_abs(j)*E_abs(k)*abs(Y(j,k))*sin(delta_plus(j)-delta_plus(k)-angle(Y(j,k))));
                else
                    sum=sum;
                end          
            C(j,i)=sum;
            end
        else
            C(j,i)=E_abs(j)*E_abs(i)*abs(Y(j,i))*sin(delta_plus(j)-delta_plus(i)-angle(Y(j,i)));
        end
    end
end
H=[C,zeros(3)];
V=eye(3);

%%% Correction:
estimatedOutput=zeros(3,1);
for i=1:3
    sum1=0;
    for j=1:5

        sum1=sum1+E_abs(i)*E_abs(j)*abs(Y(i,j))*cos(delta_(i)-delta_(j)-angle(Y(i,j))); % All angles in Radian
    end
    estimatedOutput(i)=sum1;
end

K_gain=P_*H'*(H*P_*H'+V*R*V')^-1;
estimatedStates=[delta_(1:3,1);omega_]+K_gain*(output(1:3,1)-estimatedOutput);
P_plus=(eye(6)-K_gain*H)*P_;

== matlab function Discrete_EKF_2FMU/Power System/FMU3/MATLAB Function1 ==
  data: y input; u input; dy output; P_m input; P_e output
%% This function formulates the dynamic model of the third synchronous machine in IEEE-14 bus test system
%% y is the state vector related to this Genrator, u is vector of all generators angles (delta), and P-m is Mechanical power injected to this machine
%% dy is the derivative of y which is calculated in this function and P-e is the electrical power which is calculated in this function
function [dy,P_e] = fcn(y,u,P_m) 
dy=zeros(2,1);
P_e=0;
%%%%%%%Generators and network parameters (they can be defined as global
%%%%%%%parameters because they are fixed for all generators)%%%%%%%%%%%
N_SG=5;
X_d=[0.898 1.05 1.05 1.25 1.25];
Vol_mag=[1.06 1.045 1.01 1.011981 1.049336 1.016012 1.07 1.09 1.032756 1.03177 1.04708 1.053428 1.046967 1.020701];
P_Gen=[2.32 0.4 0 0 0];
Q_Gen=[0 0.424 0 0 0];
VOl_mag_Gen=[Vol_mag(1) Vol_mag(2) Vol_mag(3) Vol_mag(6) Vol_mag(8)];
M=[3.52e-3 0.436e-3 0.436e-3 1.406e-4 1.406e-4];
D=[2 2 2 2 2];
Y=[0.1017-2.4199i, 0.0096+0.9097i, -0.0567+0.5006i, -0.0322+0.4973i, -0.0186+0.5531i; 0.0096+0.9097i, 0.1375-3.5521i, -0.0574+0.9568i, -0.0437+0.8608i, ...
    -0.0395+0.8903i; -0.0567+0.5006i, -0.0574+0.9568i, 0.2630-2.9134i, -0.0640+0.8148i, -0.0791+0.6968i; -0.0322+0.4973i, -0.0437+0.8608i, -0.0640+0.8148i,...
    0.1156-3.0762i, 0.0303+0.9547i; -0.0186+0.5531i, -0.0395+0.8903i, -0.0791+0.6968i, 0.0303+0.9547i, 0.1117-3.0513i];
% [v_r, v_i]=pol2cart(Degrre_Gen,Vol_mag_Gen);

E_abs=zeros(5,1);
for i=1:5
    %     delta0(i)=angle(VOl_mag_Gen(i)+Q_Gen(i).*X_d(i)./VOl_mag_Gen(i) + 1i*P_Gen(i).*X_d(i)./VOl_mag_Gen(i))+Degrre_Gen(i);
    E_abs(i)=abs(VOl_mag_Gen(i)+Q_Gen(i).*X_d(i)./VOl_mag_Gen(i) + 1i*P_Gen(i).*X_d(i)./VOl_mag_Gen(i));
end
%%%%%%%%%%%%%%%%%%%%%%%%%%
delta=u(1:5);
sum1=0; %% local parameter
for j=1:N_SG

    sum1=sum1+E_abs(3)*E_abs(j)*abs(Y(3,j))*cos(delta(3)-delta(j)-angle(Y(3,j))); % All angles in Radian
end

P_e=sum1;

P_e=sum1;  % Second output (which is send to the estimation part)

dy(1)=y(2); %first entry of the function output

dy(2) =(1/M(3))*(P_m-P_e-D(3)*y(2));  %Second entry of the function output
